simulink model "lqrcontrol_1"  (R2017b)
settings: Solver=ode45  StartTime=0.0  StopTime=2500  FixedStep=0.01  MaxStep=0.01  RelTol=1e-3
values from neighbouring files (symbols this model uses):
  azi0 = 10*pi/180    (= 0.174532925199)    [plot_1.m]    (also in plot_b1.m = 0.698131700798)
  bz =     [bz.mat]
  cd0 = -0.03795    [calcu_hv.m]    (also in constant_sim.m; dydt.m; dydt1.m)
  cd1 = 0.001944*57.3^2    (= 6.38271576)    [calcu_hv.m]    (also in constant_sim.m; dydt.m; dydt1.m)
  cd2 = -0.05119/340    (= -0.000150558823529)    [calcu_hv.m]    (also in constant_sim.m; dydt.m; dydt1.m)
  cl0 = -0.998    [calcu_hv.m]    (also in constant_sim.m; dydt.m; dydt1.m)
  cl1 = 0.07412*57.3    (= 4.247076)    [calcu_hv.m]    (also in constant_sim.m; dydt.m; dydt1.m)
  cl2 = 0.0017/340    (= 5e-06)    [calcu_hv.m]    (also in constant_sim.m; dydt.m; dydt1.m)
  delta_d = 0    [constant_sim.m]
  delta_l = 0    [constant_sim.m]
  fpa0 = -2*pi/180    (= -0.0349065850399)    [plot_1.m]    (also in plot_b1.m)
  hs = 7320    [calcu_hv.m]    (also in constant_sim.m; dydt.m; dydt1.m)
  K1 = reshape(K(1,:,:),3,length(bz.V)).'    [calcu_A_B1.m]
  K2 = reshape(K(2,:,:),3,length(bz.V)).'    [calcu_A_B1.m]
  lat0 = 0    [plot_1.m]    (also in plot_b1.m)
  lon0 = 0    [plot_1.m]    (also in plot_b1.m)
  m = auxdata.mass    [bianjie1.m]    (also in calcu_hv.m = 498.95; constant_sim.m = 498.95; dydt.m = 498.95; dydt1.m = 498.95)
  mu = g0*Re^2    (= 3.9823350434e+14)    [calcu_hv.m]    (also in constant_sim.m; dydt.m; dydt1.m)
  r0 = 100000+6371393    (= 6471393)    [main_1.m]    (also in main_2.m; plot_1.m = Re+90000; plot_b1.m = Re+100000)
  Re = 6371393    [calcu_hv.m]    (also in constant_sim.m; dydt.m; dydt1.m)
  rho0 = 1.225    [calcu_hv.m]    (also in constant_sim.m; dydt.m; dydt1.m)
  S = auxdata.S    [bianjie1.m]    (also in calcu_hv.m = 0.113; constant_sim.m = 0.113; dydt.m = 0.113; dydt1.m = 0.113)
  V0 = 7900    [main_1.m]    (also in main_2.m; plot_1.m; plot_b1.m)
settings Model: NumberOfSteps=1000  Creator=ztyab  LastModifiedBy=ztyab
settings DataIOCC: SaveFormat=Array

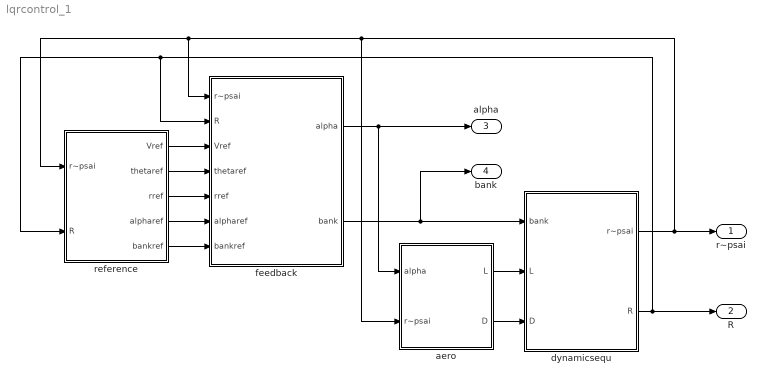
== system lqrcontrol_1 ==
  aero : Subsystem
  dynamicsequ : Subsystem
  feedback : Subsystem
  reference : Subsystem
  r~psai : Outport
  R : Outport  Port=2
  alpha : Outport  Port=3
  bank : Outport  Port=4
  wires:
  aero/2(D) -> dynamicsequ/3(D)
  aero/1(L) -> dynamicsequ/2(L)
  dynamicsequ/1(r~psai) -> feedback/1(r~psai), reference/1(r~psai), aero/2(r~psai), r~psai/1
  dynamicsequ/2(R) -> feedback/2(R), reference/2(R), R/1
  reference/5(bankref) -> feedback/7(bankref)
  reference/4(alpharef) -> feedback/6(alpharef)
  reference/3(rref) -> feedback/5(rref)
  reference/2(thetaref) -> feedback/4(thetaref)
  reference/1(Vref) -> feedback/3(Vref)
  feedback/1(alpha) -> aero/1(alpha), alpha/1
  feedback/2(bank) -> dynamicsequ/1(bank), bank/1

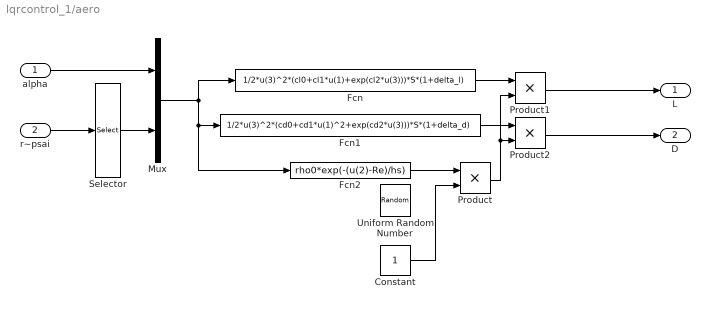
== system lqrcontrol_1/aero ==
  alpha : Inport
  r~psai : Inport  Port=2
  Constant : Constant
  Fcn : Fcn  Expr=1/2*u(3)^2*(cl0+cl1*u(1)+exp(cl2*u(3)))*S*(1+delta_l)
  Fcn1 : Fcn  Expr=1/2*u(3)^2*(cd0+cd1*u(1)^2+exp(cd2*u(3)))*S*(1+delta_d)
  Fcn2 : Fcn  Expr=rho0*exp(-(u(2)-Re)/hs)
  Mux : Mux  Inputs=2
  Product : Product
  Product1 : Product
  Product2 : Product
  Selector : Selector  InputPortWidth=6  IndexOptions=Index vector (dialog)  Indices=[1 4]  OutputSizes=1
  Uniform Random Number : UniformRandomNumber  Minimum=0.75  Maximum=1.25  SampleTime=0.5
  L : Outport
  D : Outport  Port=2
  wires:
  Mux/1 -> Fcn1/1, Fcn2/1, Fcn/1
  alpha/1 -> Mux/1
  r~psai/1 -> Selector/1
  Selector/1 -> Mux/2
  Fcn2/1 -> Product/1
  Product/1 -> Product1/2, Product2/2
  Fcn/1 -> Product1/1
  Fcn1/1 -> Product2/1
  Product1/1 -> L/1
  Product2/1 -> D/1
  Constant/1 -> Product/2

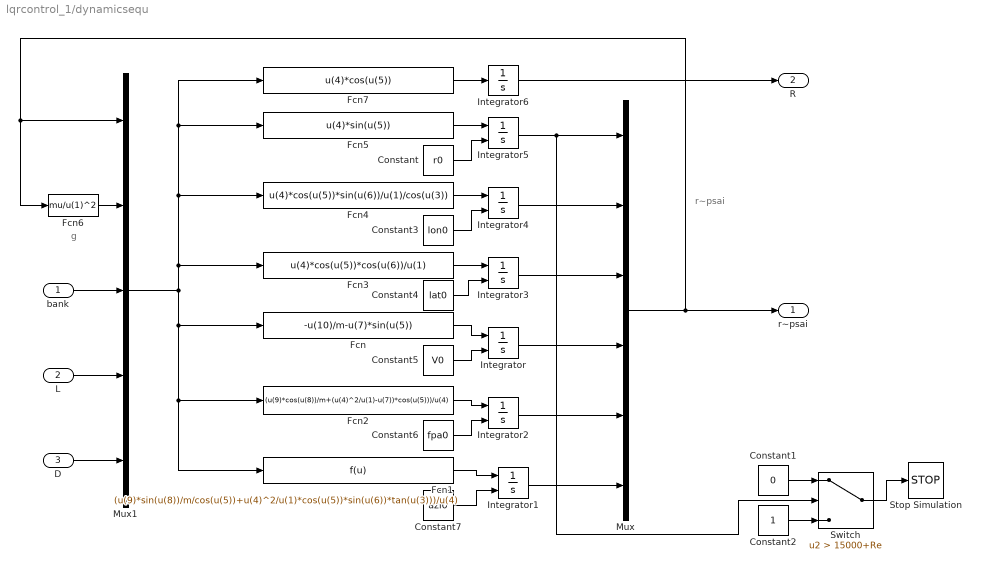
== system lqrcontrol_1/dynamicsequ ==
  note: g
  note: r~psai
  bank : Inport
  L : Inport  Port=2
  D : Inport  Port=3
  Constant : Constant  Value=r0
  Constant1 : Constant  Value=0
  Constant2 : Constant
  Constant3 : Constant  Value=lon0
  Constant4 : Constant  Value=lat0
  Constant5 : Constant  Value=V0
  Constant6 : Constant  Value=fpa0
  Constant7 : Constant  Value=azi0
  Fcn : Fcn  Expr=-u(10)/m-u(7)*sin(u(5))
  Fcn1 : Fcn  Expr=(u(9)*sin(u(8))/m/cos(u(5))+u(4)^2/u(1)*cos(u(5))*sin(u(6))*tan(u(3)))/u(4)
  Fcn2 : Fcn  Expr=(u(9)*cos(u(8))/m+(u(4)^2/u(1)-u(7))*cos(u(5)))/u(4)
  Fcn3 : Fcn  Expr=u(4)*cos(u(5))*cos(u(6))/u(1)
  Fcn4 : Fcn  Expr=u(4)*cos(u(5))*sin(u(6))/u(1)/cos(u(3))
  Fcn5 : Fcn  Expr=u(4)*sin(u(5))
  Fcn6 : Fcn  Expr=mu/u(1)^2
  Fcn7 : Fcn  Expr=u(4)*cos(u(5))
  Integrator : Integrator  InitialConditionSource=external  InitialCondition=7500
  Integrator1 : Integrator  InitialConditionSource=external  InitialCondition=10*pi/180
  Integrator2 : Integrator  InitialConditionSource=external  InitialCondition=-2/180*pi
  Integrator3 : Integrator  InitialConditionSource=external
  Integrator4 : Integrator  InitialConditionSource=external
  Integrator5 : Integrator  InitialConditionSource=external  InitialCondition=95000+6371393
  Integrator6 : Integrator
  Mux : Mux  Inputs=6
  Mux1 : Mux  Inputs=5
  Stop Simulation : Stop
  Switch : Switch  Criteria=u2 > Threshold  Threshold=15000+Re
  r~psai : Outport
  R : Outport  Port=2
  wires:
  Fcn6/1 -> Mux1/2
  Mux/1 -> Fcn6/1, Mux1/1, r~psai/1
  Fcn1/1 -> Integrator1/1
  Integrator1/1 -> Mux/6
  Fcn2/1 -> Integrator2/1
  Integrator4/1 -> Mux/2
  Fcn/1 -> Integrator/1
  Integrator2/1 -> Mux/5
  Fcn4/1 -> Integrator4/1
  Integrator3/1 -> Mux/3
  Fcn3/1 -> Integrator3/1
  Integrator/1 -> Mux/4
  Fcn5/1 -> Integrator5/1
  L/1 -> Mux1/4
  D/1 -> Mux1/5
  bank/1 -> Mux1/3
  Mux1/1 -> Fcn1/1, Fcn2/1, Fcn/1, Fcn4/1, Fcn7/1, Fcn5/1, Fcn3/1
  Fcn7/1 -> Integrator6/1
  Integrator6/1 -> R/1
  Constant2/1 -> Switch/3
  Constant1/1 -> Switch/1
  Switch/1 -> Stop Simulation/1
  Constant/1 -> Integrator5/2
  Constant3/1 -> Integrator4/2
  Constant4/1 -> Integrator3/2
  Constant5/1 -> Integrator/2
  Constant6/1 -> Integrator2/2
  Constant7/1 -> Integrator1/2
  Integrator5/1 -> Switch/2, Mux/1

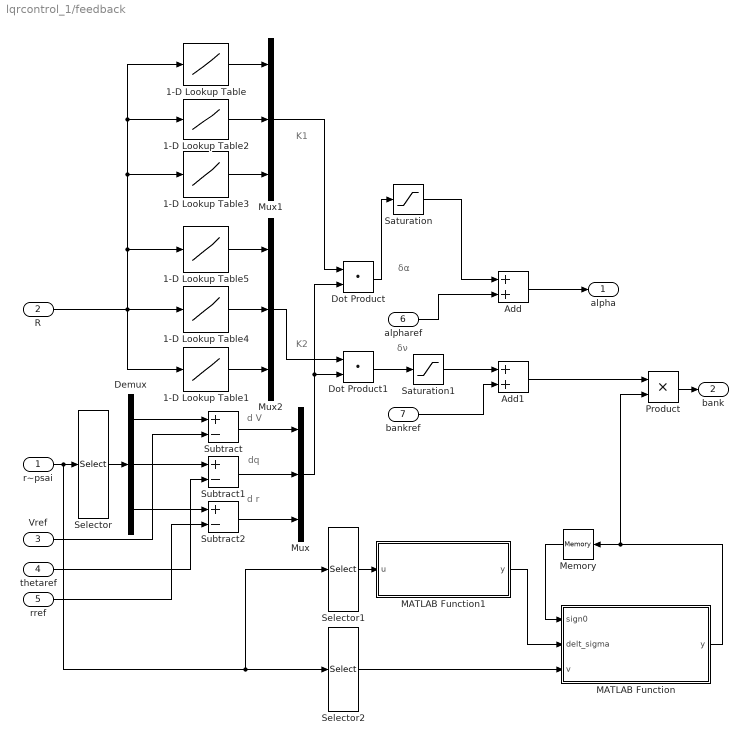
== system lqrcontrol_1/feedback ==
  note: δν
  note: δα
  note: K2
  note: K1
  note: d V
  note: d r
  note: dq
  r~psai : Inport
  R : Inport  Port=2
  Vref : Inport  Port=3
  thetaref : Inport  Port=4
  rref : Inport  Port=5
  alpharef : Inport  Port=6
  bankref : Inport  Port=7
  1-D Lookup Table : Lookup_n-D  NumberOfTableDimensions=1  BreakpointsForDimension1=bz.R  Table=-K1(:,1)  InterpMethod=Cubic spline  ExtrapMethod=Cubic spline  InternalRulePriority=Speed  RndMeth=Simplest  InputSameDT=on
  1-D Lookup Table1 : Lookup_n-D  NumberOfTableDimensions=1  BreakpointsForDimension1=bz.R  Table=-K2(:,3)  InterpMethod=Cubic spline  ExtrapMethod=Cubic spline  InternalRulePriority=Speed  RndMeth=Simplest  InputSameDT=on
  1-D Lookup Table2 : Lookup_n-D  NumberOfTableDimensions=1  BreakpointsForDimension1=bz.R  Table=-K1(:,2)  InterpMethod=Cubic spline  ExtrapMethod=Cubic spline  InternalRulePriority=Speed  RndMeth=Simplest  InputSameDT=on
  1-D Lookup Table3 : Lookup_n-D  NumberOfTableDimensions=1  BreakpointsForDimension1=bz.R  Table=-K1(:,3)  InterpMethod=Cubic spline  ExtrapMethod=Cubic spline  InternalRulePriority=Speed  RndMeth=Simplest  InputSameDT=on
  1-D Lookup Table4 : Lookup_n-D  NumberOfTableDimensions=1  BreakpointsForDimension1=bz.R  Table=-K2(:,2)  InterpMethod=Cubic spline  ExtrapMethod=Cubic spline  InternalRulePriority=Speed  RndMeth=Simplest  InputSameDT=on
  1-D Lookup Table5 : Lookup_n-D  NumberOfTableDimensions=1  BreakpointsForDimension1=bz.R  Table=-K2(:,1)  InterpMethod=Cubic spline  ExtrapMethod=Cubic spline  InternalRulePriority=Speed  RndMeth=Simplest  InputSameDT=on
  Add : Sum
  Add1 : Sum
  Demux : Demux  Outputs=3
  Dot Product : DotProduct  InputSameDT=on  OutDataTypeStr=Inherit: Inherit via internal rule
  Dot Product1 : DotProduct  InputSameDT=on  OutDataTypeStr=Inherit: Inherit via internal rule
  MATLAB Function : MATLAB Function  TreatAsAtomicUnit=on
  MATLAB Function1 : MATLAB Function  TreatAsAtomicUnit=on
  Memory : Memory
  Mux : Mux  Inputs=3
  Mux1 : Mux  Inputs=3
  Mux2 : Mux  Inputs=3
  Product : Product
  Saturation : Saturate  UpperLimit=5/57.3  LowerLimit=-5/57.3
  Saturation1 : Saturate  UpperLimit=5/57.3  LowerLimit=-5/57.3
  Selector : Selector  InputPortWidth=6  IndexOptions=Index vector (dialog)  Indices=[4 5 1]  OutputSizes=1
  Selector1 : Selector  InputPortWidth=6  IndexOptions=Index vector (dialog)  Indices=[2 3 6]  OutputSizes=1
  Selector2 : Selector  InputPortWidth=6  IndexOptions=Index vector (dialog)  Indices=[4]  OutputSizes=1
  Subtract : Sum  Inputs=+-
  Subtract1 : Sum  Inputs=+-
  Subtract2 : Sum  Inputs=+-
  alpha : Outport
  bank : Outport  Port=2
  wires:
  bankref/1 -> Add1/2
  Subtract/1 -> Mux/1
  Subtract1/1 -> Mux/2
  Demux/2 -> Subtract1/1
  Demux/3 -> Subtract2/1
  Selector/1 -> Demux/1
  thetaref/1 -> Subtract1/2
  Demux/1 -> Subtract/1
  Mux/1 -> Dot Product/2, Dot Product1/2
  Subtract2/1 -> Mux/3
  rref/1 -> Subtract2/2
  Add/1 -> alpha/1
  Dot Product/1 -> Saturation/1
  Dot Product1/1 -> Saturation1/1
  alpharef/1 -> Add/2
  1-D Lookup Table2/1 -> Mux1/2
  1-D Lookup Table/1 -> Mux1/1
  1-D Lookup Table3/1 -> Mux1/3
  Mux1/1 -> Dot Product/1
  1-D Lookup Table4/1 -> Mux2/2
  1-D Lookup Table1/1 -> Mux2/3
  1-D Lookup Table5/1 -> Mux2/1
  Mux2/1 -> Dot Product1/1
  Memory/1 -> MATLAB Function/1(sign0)
  Selector2/1 -> MATLAB Function/3(v)
  MATLAB Function1/1(y) -> MATLAB Function/2(delt_sigma)
  r~psai/1 -> Selector2/1, Selector1/1, Selector/1
  Saturation/1 -> Add/1
  MATLAB Function/1(y) -> Product/2, Memory/1
  Saturation1/1 -> Add1/1
  Add1/1 -> Product/1
  Product/1 -> bank/1
  Selector1/1 -> MATLAB Function1/1(u)
  R/1 -> 1-D Lookup Table1/1, 1-D Lookup Table5/1, 1-D Lookup Table2/1, 1-D Lookup Table/1, 1-D Lookup Table3/1, 1-D Lookup Table4/1
  Vref/1 -> Subtract/2

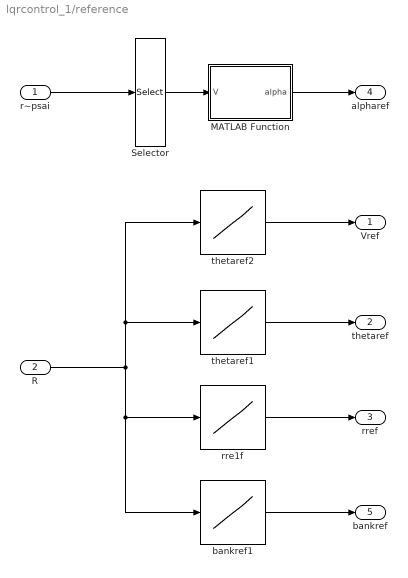
== system lqrcontrol_1/reference ==
  r~psai : Inport
  R : Inport  Port=2
  MATLAB Function : MATLAB Function  TreatAsAtomicUnit=on
  Selector : Selector  InputPortWidth=6  IndexOptions=Index vector (dialog)  Indices=[4]  OutputSizes=1
  bankref1 : Lookup_n-D  NumberOfTableDimensions=1  BreakpointsForDimension1=bz.R  Table=bz.nu  InterpMethod=Cubic spline  ExtrapMethod=Cubic spline  InternalRulePriority=Speed  RndMeth=Simplest  InputSameDT=on
  rre1f : Lookup_n-D  NumberOfTableDimensions=1  BreakpointsForDimension1=bz.R  Table=bz.r  InterpMethod=Cubic spline  ExtrapMethod=Cubic spline  InternalRulePriority=Speed  RndMeth=Simplest  InputSameDT=on
  thetaref1 : Lookup_n-D  NumberOfTableDimensions=1  BreakpointsForDimension1=bz.R  Table=bz.theta  InterpMethod=Cubic spline  ExtrapMethod=Cubic spline  InternalRulePriority=Speed  RndMeth=Simplest  InputSameDT=on
  thetaref2 : Lookup_n-D  NumberOfTableDimensions=1  BreakpointsForDimension1=bz.R  Table=bz.V  InterpMethod=Cubic spline  ExtrapMethod=Cubic spline  InternalRulePriority=Speed  RndMeth=Simplest  InputSameDT=on
  Vref : Outport
  thetaref : Outport  Port=2
  rref : Outport  Port=3
  alpharef : Outport  Port=4
  bankref : Outport  Port=5
  wires:
  bankref1/1 -> bankref/1
  r~psai/1 -> Selector/1
  MATLAB Function/1(alpha) -> alpharef/1
  thetaref1/1 -> thetaref/1
  Selector/1 -> MATLAB Function/1(V)
  rre1f/1 -> rref/1
  R/1 -> rre1f/1, bankref1/1, thetaref1/1, thetaref2/1
  thetaref2/1 -> Vref/1

== matlab function lqrcontrol_1/feedback/MATLAB Function1 ==
  data: u input; y output
function y = fcn(u)
lambda=u(1);
phi=u(2);
sigma=u(3);
lambdaf=38.62*pi/180;
phif=21.83*pi/180;
if phi>phif
    sigma_t=pi-asin(cos(phif)*sin(lambdaf-lambda)/sin(acos(sin(phif)*sin(phi)+cos(phif)*cos(phi)*cos(lambdaf-lambda))));
else
    sigma_t=asin(cos(phif)*sin(lambdaf-lambda)/sin(acos(sin(phif)*sin(phi)+cos(phif)*cos(phi)*cos(lambdaf-lambda))));
end
y=sigma-sigma_t;
end

== matlab function lqrcontrol_1/reference/MATLAB Function ==
  data: V input; alpha output
function alpha = calcu_alpha(V)

v1=6500;
v2=5000;
alpha0=20*pi/180;
alphaf=10*pi/180;
alpha=(alpha0.*(V>v1)+((V-v1)*(alphaf-alpha0)/(v2-v1)+alpha0).*(V<=v1&V>=v2)+alphaf.*(V<v2));

end

== matlab function lqrcontrol_1/feedback/MATLAB Function ==
  data: sign0 input; y output; delt_sigma input; v input
function y = fcn(sign0,delt_sigma,v)

%#codegen
delt_sigma1=10/180*pi;
delt_sigma2=20/180*pi;
delt_sigma3=5/180*pi;
if (v>=5000)
    if (delt_sigma>delt_sigma1)
        sign=-1;
    elseif (delt_sigma<=delt_sigma1)&&(delt_sigma>=-delt_sigma1)
        sign=sign0;
    else 
        sign=1;
    end
elseif (4000<=v&v<5000)
    if (delt_sigma>delt_sigma2)
        sign=-1;
    elseif (delt_sigma<=delt_sigma2)&&(delt_sigma>=-delt_sigma2)
        sign=sign0;
    else 
        sign=1;
    end
elseif (3000<=v&&v<4000)
    delt=delt_sigma3+(delt_sigma2-delt_sigma3)/(4000-3000)*(v-3000);
    if (delt_sigma>delt)
        sign=-1;
    elseif (delt_sigma<=delt)&&(delt_sigma>=-delt)
        sign=sign0;
    else 
        sign=1;
    end  
else
    if (delt_sigma>delt_sigma3)
        sign=-1;
    elseif (delt_sigma<=delt_sigma3)&&(delt_sigma>=-delt_sigma3)
        sign=sign0;
    else 
        sign=1;
    end  
end
if(sign0==0)
    sign=1;
end
y =sign;
end
